simulink model "Nanosatellite"  (Simulink 10.1)
settings: Solver=FixedStepAuto  StartTime=0.0  StopTime=5  FixedStep=1e-2  RelTol=1e-3
undefined symbols (not defined in the file): a1, a2, a3, K, K1, K2, u10, u20
settings Model: Creator=NAOUE  LastModifiedBy=NAOUE
settings DataIOCC: SaveFormat=Dataset  ReturnWorkspaceOutputs=on
settings OptimizationCC: LifeSpan=auto
settings DebuggingCC: UnderspecifiedInitializationDetection=Simplified  MergeDetectMultiDrivingBlocksExec=error  SFUnexpectedBacktrackingDiag=error  SFNoUnconditionalDefaultTransitionDiag=error  SFExecutionAtInitializationDiag=warning  ArithmeticOperatorsInVariantConditions=error
settings HardwareCC: ProdBitPerPointer=64  ProdBitPerSizeT=64  ProdBitPerPtrDiffT=64  ProdLargestAtomicFloat=Float  ProdIntDivRoundTo=Zero  ProdEndianess=LittleEndian  ProdWordSize=64  ProdHWDeviceType=Intel->x86-64 (Windows64)
settings ModelReferenceCC: PropagateSignalLabelsOutOfModel=on
settings SFSimCC: SimUseLocalCustomCode=on  CustomCodeUndefinedFunction=FilterOut
settings RTWCC: RTWUseLocalCustomCode=on
settings CodeAppCC: StateflowObjectComments=off
settings GRTTargetCC: TargetLangStandard=C99 (ISO)  CombineOutputUpdateFcns=on  GRTInterface=off
settings ConfigComp: CovMetricSettings=dwe  CovHtmlReporting=off  CovSaveCumulativeToWorkspaceVar=off  CovSaveSingleToWorkspaceVar=off  CovExternalEMLEnable=on

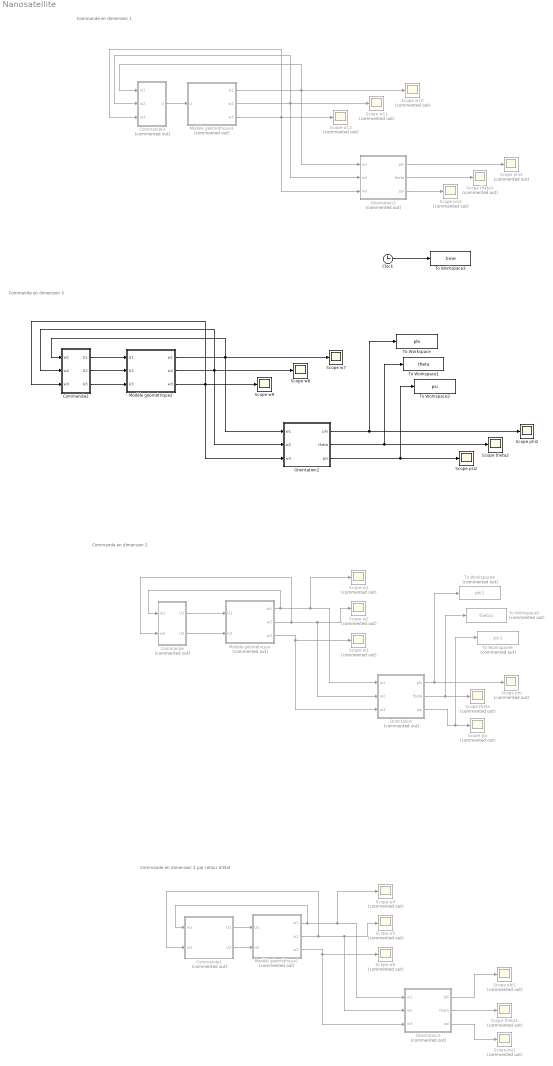
== system Nanosatellite ==
  note: Commande en dimension 2 par retour d'état
  note: Commande en dimension 2
  note: Commande en dimension 1
  note: Commande en dimension 3
  Clock : Clock
  Commande : Subsystem  Commented=on
  Commande1 : Subsystem  Commented=on
  Commande2 : Subsystem
  Commande3 : Subsystem  Commented=on
  Modèle géométrique : Subsystem  Commented=on
  Modèle géométrique1 : Subsystem  Commented=on
  Modèle géométrique2 : Subsystem
  Modèle géométrique3 : Subsystem  Commented=on
  Orientation : Subsystem  Commented=on
  Orientation1 : Subsystem  Commented=on
  Orientation2 : Subsystem
  Orientation3 : Subsystem  Commented=on
  Scope phi : Scope  Commented=on
  Scope phi1 : Scope  Commented=on
  Scope phi2 : Scope
  Scope phi3 : Scope  Commented=on
  Scope psi : Scope  Commented=on
  Scope psi1 : Scope  Commented=on
  Scope psi2 : Scope
  Scope psi3 : Scope  Commented=on
  Scope theta : Scope  Commented=on
  Scope theta1 : Scope  Commented=on
  Scope theta2 : Scope
  Scope theta3 : Scope  Commented=on
  Scope w{1..6,10..12} (9 alike) : Scope  Commented=on
  Scope w7 : Scope
  Scope w8 : Scope
  Scope w9 : Scope
  To Workspace : ToWorkspace  VariableName=phi  SampleTime=-1
  To Workspace1 : ToWorkspace  VariableName=theta  SampleTime=-1
  To Workspace2 : ToWorkspace  VariableName=psi  SampleTime=-1
  To Workspace3 : ToWorkspace  VariableName=time  SampleTime=-1
  To Workspace4 : ToWorkspace  Commented=on  VariableName=phi1  SampleTime=-1
  To Workspace5 : ToWorkspace  Commented=on  VariableName=theta1  SampleTime=-1
  To Workspace6 : ToWorkspace  Commented=on  VariableName=psi1  SampleTime=-1
  wires:
  Modèle géométrique/3(w3) -> Orientation/3(w3), Scope w3/1
  Commande/1(U1) -> Modèle géométrique/1(U1)
  Commande/2(U2) -> Modèle géométrique/2(U2)
  Modèle géométrique/1(w1) -> Commande/1(w1), Orientation/1(w1), Scope w1/1
  Modèle géométrique/2(w2) -> Commande/2(w2), Orientation/2(w2), Scope w2/1
  Modèle géométrique1/2(w2) -> Commande1/2(w2), Scope w5/1, Orientation1/2(w2)
  Modèle géométrique1/1(w1) -> Commande1/1(w1), Scope w4/1, Orientation1/1(w1)
  Commande1/2(U2) -> Modèle géométrique1/2(U2)
  Commande1/1(U1) -> Modèle géométrique1/1(U1)
  Orientation1/3(psi) -> Scope psi1/1
  Orientation1/2(theta) -> Scope theta1/1
  Orientation1/1(phi) -> Scope phi1/1
  Modèle géométrique1/3(w3) -> Scope w6/1, Orientation1/3(w3)
  Modèle géométrique2/2(w2) -> Commande2/2(w2), Scope w8/1, Orientation2/2(w2)
  Modèle géométrique2/1(w1) -> Commande2/1(w1), Scope w7/1, Orientation2/1(w1)
  Commande2/2(U2) -> Modèle géométrique2/2(U2)
  Commande2/1(U1) -> Modèle géométrique2/1(U1)
  Orientation2/3(psi) -> To Workspace2/1, Scope psi2/1
  Orientation2/2(theta) -> Scope theta2/1, To Workspace1/1
  Orientation2/1(phi) -> To Workspace/1, Scope phi2/1
  Modèle géométrique2/3(w3) -> Commande2/3(w3), Scope w9/1, Orientation2/3(w3)
  Commande2/3(U3) -> Modèle géométrique2/3(U3)
  Modèle géométrique3/3(w3) -> Orientation3/3(w3), Commande3/3(w3), Scope w12/1
  Orientation3/1(phi) -> Scope phi3/1
  Orientation3/2(theta) -> Scope theta3/1
  Orientation3/3(psi) -> Scope psi3/1
  Commande3/1(U) -> Modèle géométrique3/1(U)
  Modèle géométrique3/1(w1) -> Orientation3/1(w1), Scope w10/1, Commande3/1(w1)
  Modèle géométrique3/2(w2) -> Orientation3/2(w2), Scope w11/1, Commande3/2(w2)
  Clock/1 -> To Workspace3/1
  Orientation/1(phi) -> To Workspace4/1, Scope phi/1
  Orientation/2(theta) -> To Workspace5/1, Scope theta/1
  Orientation/3(psi) -> To Workspace6/1, Scope psi/1

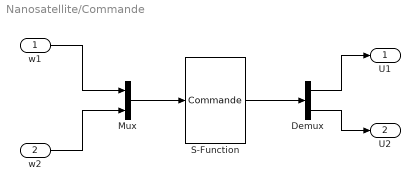
== system Nanosatellite/Commande ==
  w1 : Inport
  w2 : Inport  Port=2
  Demux : Demux  Outputs=2
  Mux : Mux  Inputs=2
  S-Function : S-Function  FunctionName=Commande  Parameters=Parametres  SFunctionDeploymentMode=off  EnableBusSupport=off
  U1 : Outport
  U2 : Outport  Port=2
  wires:
  S-Function/1 -> Demux/1
  w1/1 -> Mux/1
  Demux/1 -> U1/1
  w2/1 -> Mux/2
  Demux/2 -> U2/1
  Mux/1 -> S-Function/1

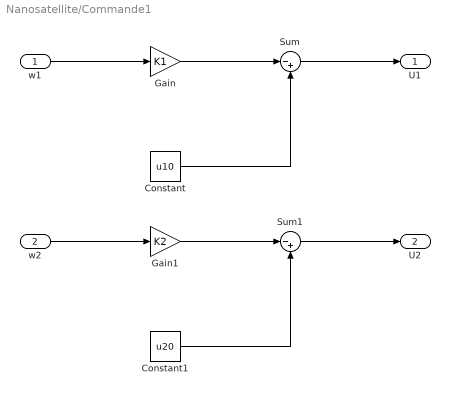
== system Nanosatellite/Commande1 ==
  w1 : Inport
  w2 : Inport  Port=2
  Constant : Constant  Value=u10
  Constant1 : Constant  Value=u20
  Gain : Gain  Gain=K1
  Gain1 : Gain  Gain=K2
  Sum : Sum  Inputs=|-+
  Sum1 : Sum  Inputs=|-+
  U1 : Outport
  U2 : Outport  Port=2
  wires:
  Gain/1 -> Sum/1
  w1/1 -> Gain/1
  Constant/1 -> Sum/2
  Sum/1 -> U1/1
  Sum1/1 -> U2/1
  Constant1/1 -> Sum1/2
  w2/1 -> Gain1/1
  Gain1/1 -> Sum1/1

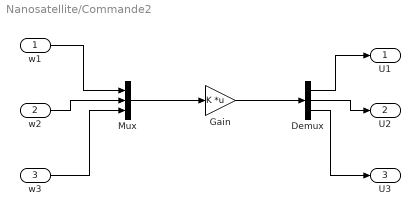
== system Nanosatellite/Commande2 ==
  w1 : Inport
  w2 : Inport  Port=2
  w3 : Inport  Port=3
  Demux : Demux  Outputs=3
  Gain : Gain  Gain=K  Multiplication=Matrix(K*u)
  Mux : Mux  Inputs=3
  U1 : Outport
  U2 : Outport  Port=2
  U3 : Outport  Port=3
  wires:
  Mux/1 -> Gain/1
  Demux/2 -> U2/1
  w2/1 -> Mux/2
  Demux/1 -> U1/1
  w1/1 -> Mux/1
  Gain/1 -> Demux/1
  w3/1 -> Mux/3
  Demux/3 -> U3/1

== system Nanosatellite/Commande3 ==
  w1 : Inport
  w2 : Inport  Port=2
  w3 : Inport  Port=3
  Mux : Mux  Inputs=3
  S-Function : S-Function  FunctionName=Commande3  SFunctionDeploymentMode=off  EnableBusSupport=off
  U : Outport
  wires:
  w3/1 -> Mux/3
  w1/1 -> Mux/1
  S-Function/1 -> U/1
  w2/1 -> Mux/2
  Mux/1 -> S-Function/1

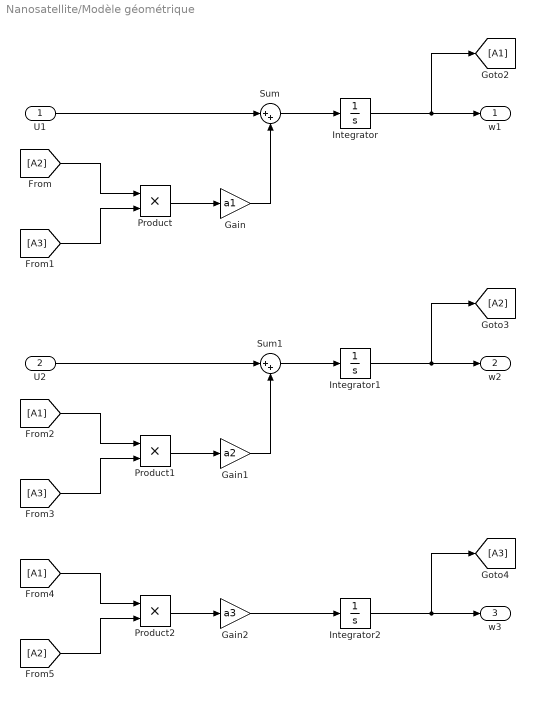
== system Nanosatellite/Modèle géométrique ==
  U1 : Inport
  U2 : Inport  Port=2
  Gain : Gain  Gain=a1
  Gain1 : Gain  Gain=a2
  Gain2 : Gain  Gain=a3
  Integrator : Integrator
  Integrator1 : Integrator
  Integrator2 : Integrator
  Product : Product
  Product1 : Product
  Product2 : Product
  Sum : Sum  Inputs=|++
  Sum1 : Sum  Inputs=|++
  w1 : Outport
  w2 : Outport  Port=2
  w3 : Outport  Port=3
  wires:
  Integrator/1 -> [A1], w1/1
  U1/1 -> Sum/1
  Sum/1 -> Integrator/1
  Gain/1 -> Sum/2
  Product/1 -> Gain/1
  [A2] -> Product/1
  [A3] -> Product/2
  [A3] -> Product1/2
  [A1] -> Product1/1
  Product1/1 -> Gain1/1
  Gain1/1 -> Sum1/2
  Sum1/1 -> Integrator1/1
  U2/1 -> Sum1/1
  Integrator1/1 -> w2/1, [A2]
  Integrator2/1 -> [A3], w3/1
  Gain2/1 -> Integrator2/1
  Product2/1 -> Gain2/1
  [A1] -> Product2/1
  [A2] -> Product2/2

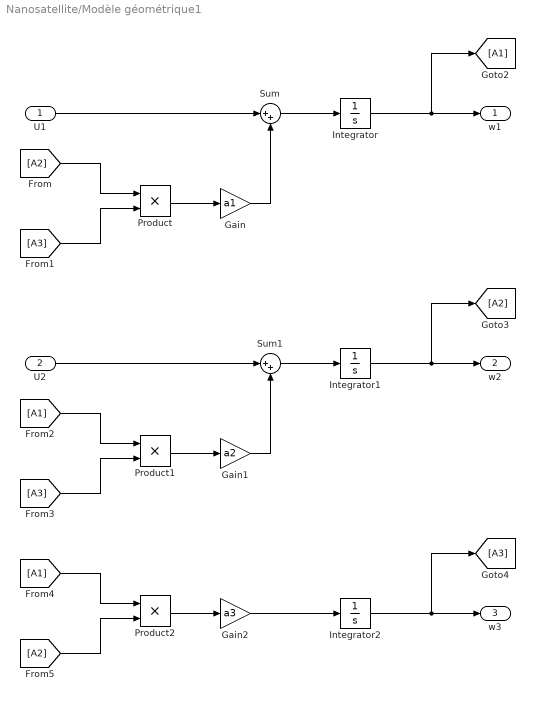
== system Nanosatellite/Modèle géométrique1 ==
  U1 : Inport
  U2 : Inport  Port=2
  Gain : Gain  Gain=a1
  Gain1 : Gain  Gain=a2
  Gain2 : Gain  Gain=a3
  Integrator : Integrator
  Integrator1 : Integrator
  Integrator2 : Integrator
  Product : Product
  Product1 : Product
  Product2 : Product
  Sum : Sum  Inputs=|++
  Sum1 : Sum  Inputs=|++
  w1 : Outport
  w2 : Outport  Port=2
  w3 : Outport  Port=3
  wires:
  [A2] -> Product2/2
  [A1] -> Product2/1
  Product2/1 -> Gain2/1
  Gain2/1 -> Integrator2/1
  Integrator2/1 -> w3/1, [A3]
  Integrator1/1 -> [A2], w2/1
  U2/1 -> Sum1/1
  Sum1/1 -> Integrator1/1
  Gain1/1 -> Sum1/2
  Product1/1 -> Gain1/1
  [A1] -> Product1/1
  [A3] -> Product1/2
  [A3] -> Product/2
  [A2] -> Product/1
  Product/1 -> Gain/1
  Gain/1 -> Sum/2
  Sum/1 -> Integrator/1
  U1/1 -> Sum/1
  Integrator/1 -> w1/1, [A1]

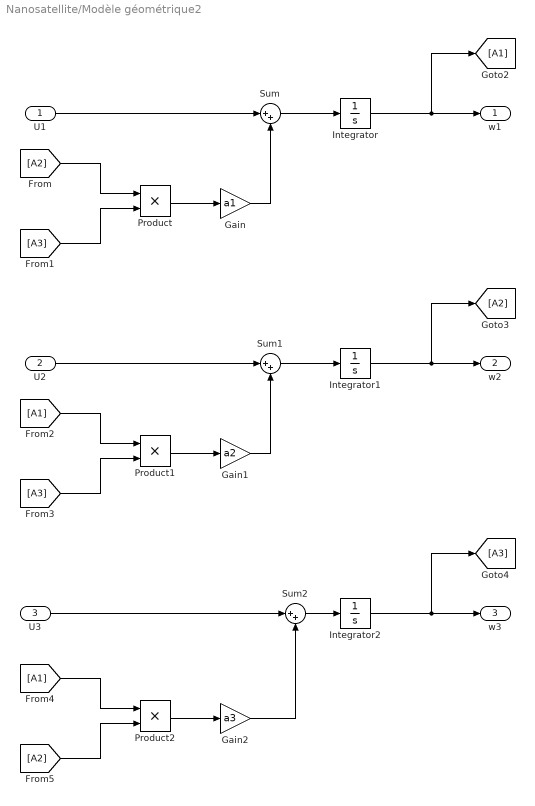
== system Nanosatellite/Modèle géométrique2 ==
  U1 : Inport
  U2 : Inport  Port=2
  U3 : Inport  Port=3
  Gain : Gain  Gain=a1
  Gain1 : Gain  Gain=a2
  Gain2 : Gain  Gain=a3
  Integrator : Integrator  InitialCondition=0.1
  Integrator1 : Integrator  InitialCondition=0.1
  Integrator2 : Integrator  InitialCondition=0.2
  Product : Product
  Product1 : Product
  Product2 : Product
  Sum : Sum  Inputs=|++
  Sum1 : Sum  Inputs=|++
  Sum2 : Sum  Inputs=|++
  w1 : Outport
  w2 : Outport  Port=2
  w3 : Outport  Port=3
  wires:
  Integrator/1 -> [A1], w1/1
  U1/1 -> Sum/1
  Sum/1 -> Integrator/1
  Gain/1 -> Sum/2
  Product/1 -> Gain/1
  [A2] -> Product/1
  [A3] -> Product/2
  [A3] -> Product1/2
  [A1] -> Product1/1
  Product1/1 -> Gain1/1
  Gain1/1 -> Sum1/2
  Sum1/1 -> Integrator1/1
  U2/1 -> Sum1/1
  Integrator1/1 -> w2/1, [A2]
  Integrator2/1 -> [A3], w3/1
  Product2/1 -> Gain2/1
  [A1] -> Product2/1
  [A2] -> Product2/2
  U3/1 -> Sum2/1
  Gain2/1 -> Sum2/2
  Sum2/1 -> Integrator2/1

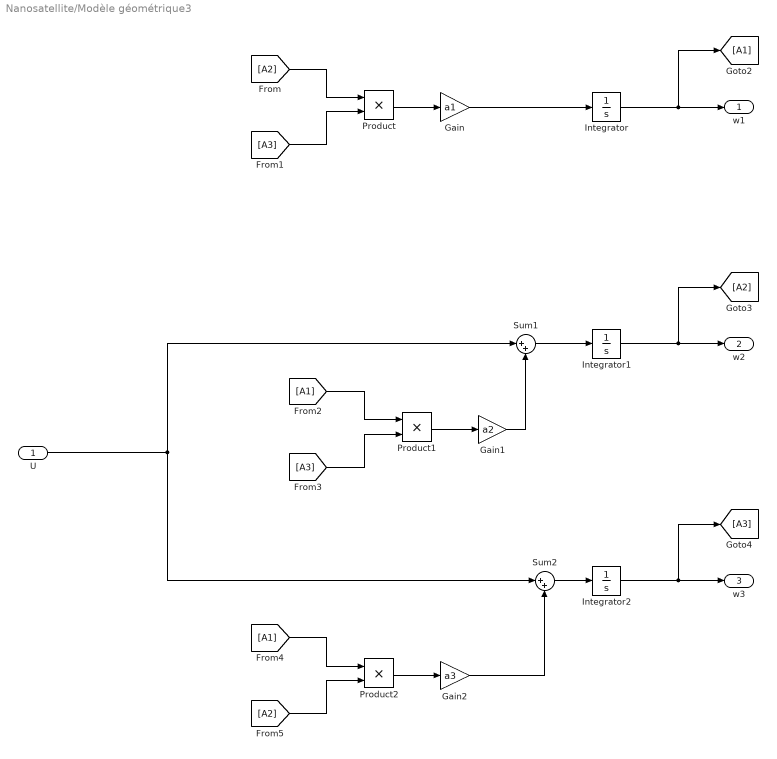
== system Nanosatellite/Modèle géométrique3 ==
  U : Inport
  Gain : Gain  Gain=a1
  Gain1 : Gain  Gain=a2
  Gain2 : Gain  Gain=a3
  Integrator : Integrator  InitialCondition=0.001
  Integrator1 : Integrator
  Integrator2 : Integrator
  Product : Product
  Product1 : Product
  Product2 : Product
  Sum1 : Sum  Inputs=|++
  Sum2 : Sum  Inputs=|++
  w1 : Outport
  w2 : Outport  Port=2
  w3 : Outport  Port=3
  wires:
  Sum2/1 -> Integrator2/1
  Gain2/1 -> Sum2/2
  [A2] -> Product2/2
  [A1] -> Product2/1
  Product2/1 -> Gain2/1
  Integrator2/1 -> w3/1, [A3]
  Integrator1/1 -> [A2], w2/1
  Sum1/1 -> Integrator1/1
  Gain1/1 -> Sum1/2
  Product1/1 -> Gain1/1
  [A1] -> Product1/1
  [A3] -> Product1/2
  [A3] -> Product/2
  [A2] -> Product/1
  Product/1 -> Gain/1
  Gain/1 -> Integrator/1
  Integrator/1 -> w1/1, [A1]
  U/1 -> Sum1/1, Sum2/1

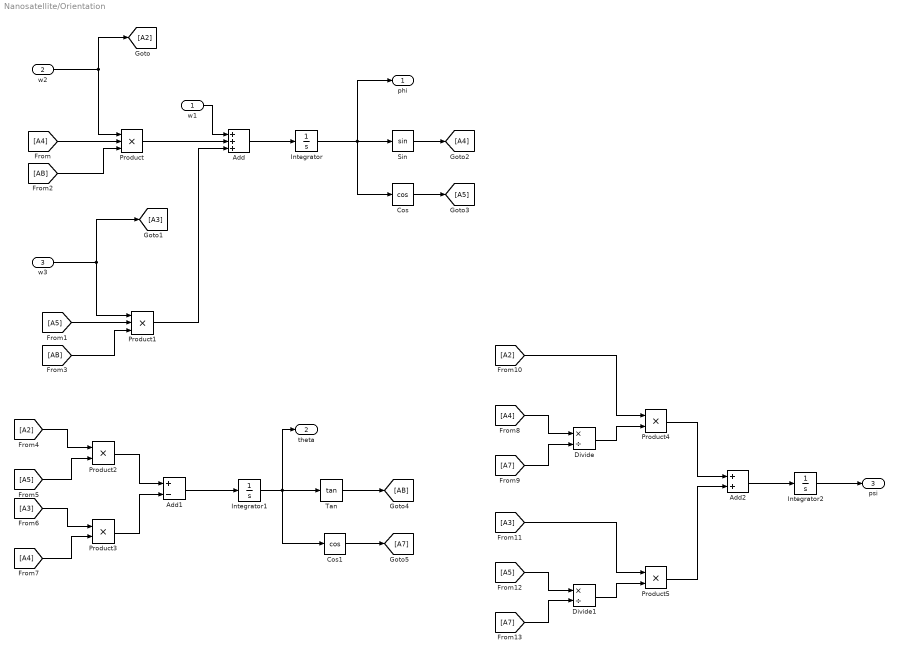
== system Nanosatellite/Orientation ==
  w1 : Inport
  w2 : Inport  Port=2
  w3 : Inport  Port=3
  Add : Sum  Inputs=+++
  Add1 : Sum  Inputs=+-
  Add2 : Sum
  Cos : Trigonometry  Operator=cos
  Cos1 : Trigonometry  Operator=cos
  Divide : Product  Inputs=*/
  Divide1 : Product  Inputs=*/
  Integrator : Integrator
  Integrator1 : Integrator
  Integrator2 : Integrator
  Product : Product  Inputs=3
  Product1 : Product  Inputs=3
  Product{2..5} (4 alike) : Product
  Sin : Trigonometry
  Tan : Trigonometry  Operator=tan
  phi : Outport
  theta : Outport  Port=2
  psi : Outport  Port=3
  wires:
  [A4] -> Product/2
  [AB] -> Product/3
  w2/1 -> [A2], Product/1
  Product/1 -> Add/2
  w1/1 -> Add/1
  Add/1 -> Integrator/1
  w3/1 -> Product1/1, [A3]
  [AB] -> Product1/3
  [A5] -> Product1/2
  Product1/1 -> Add/3
  Integrator/1 -> phi/1, Cos/1, Sin/1
  Sin/1 -> [A4]
  Cos/1 -> [A5]
  [A2] -> Product2/1
  [A5] -> Product2/2
  [A4] -> Product3/2
  [A3] -> Product3/1
  Product2/1 -> Add1/1
  Product3/1 -> Add1/2
  Add1/1 -> Integrator1/1
  Integrator1/1 -> theta/1, Cos1/1, Tan/1
  Tan/1 -> [AB]
  Cos1/1 -> [A7]
  [A7] -> Divide/2
  [A4] -> Divide/1
  [A2] -> Product4/1
  Divide/1 -> Product4/2
  Divide1/1 -> Product5/2
  [A3] -> Product5/1
  [A5] -> Divide1/1
  [A7] -> Divide1/2
  Product4/1 -> Add2/1
  Product5/1 -> Add2/2
  Add2/1 -> Integrator2/1
  Integrator2/1 -> psi/1

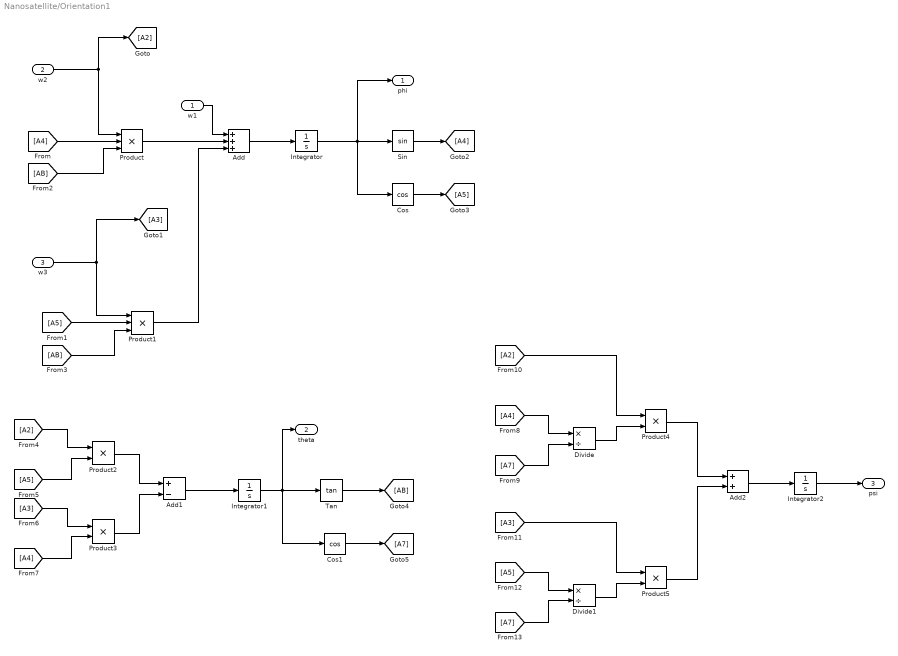
== system Nanosatellite/Orientation1 ==
  w1 : Inport
  w2 : Inport  Port=2
  w3 : Inport  Port=3
  Add : Sum  Inputs=+++
  Add1 : Sum  Inputs=+-
  Add2 : Sum
  Cos : Trigonometry  Operator=cos
  Cos1 : Trigonometry  Operator=cos
  Divide : Product  Inputs=*/
  Divide1 : Product  Inputs=*/
  Integrator : Integrator
  Integrator1 : Integrator
  Integrator2 : Integrator
  Product : Product  Inputs=3
  Product1 : Product  Inputs=3
  Product{2..5} (4 alike) : Product
  Sin : Trigonometry
  Tan : Trigonometry  Operator=tan
  phi : Outport
  theta : Outport  Port=2
  psi : Outport  Port=3
  wires:
  Integrator2/1 -> psi/1
  Add2/1 -> Integrator2/1
  Product5/1 -> Add2/2
  Product4/1 -> Add2/1
  [A7] -> Divide1/2
  [A5] -> Divide1/1
  [A3] -> Product5/1
  Divide1/1 -> Product5/2
  Divide/1 -> Product4/2
  [A2] -> Product4/1
  [A4] -> Divide/1
  [A7] -> Divide/2
  Cos1/1 -> [A7]
  Tan/1 -> [AB]
  Integrator1/1 -> Tan/1, Cos1/1, theta/1
  Add1/1 -> Integrator1/1
  Product3/1 -> Add1/2
  Product2/1 -> Add1/1
  [A3] -> Product3/1
  [A4] -> Product3/2
  [A5] -> Product2/2
  [A2] -> Product2/1
  Cos/1 -> [A5]
  Sin/1 -> [A4]
  Integrator/1 -> Sin/1, Cos/1, phi/1
  Product1/1 -> Add/3
  [A5] -> Product1/2
  [AB] -> Product1/3
  w3/1 -> [A3], Product1/1
  Add/1 -> Integrator/1
  w1/1 -> Add/1
  Product/1 -> Add/2
  w2/1 -> Product/1, [A2]
  [AB] -> Product/3
  [A4] -> Product/2

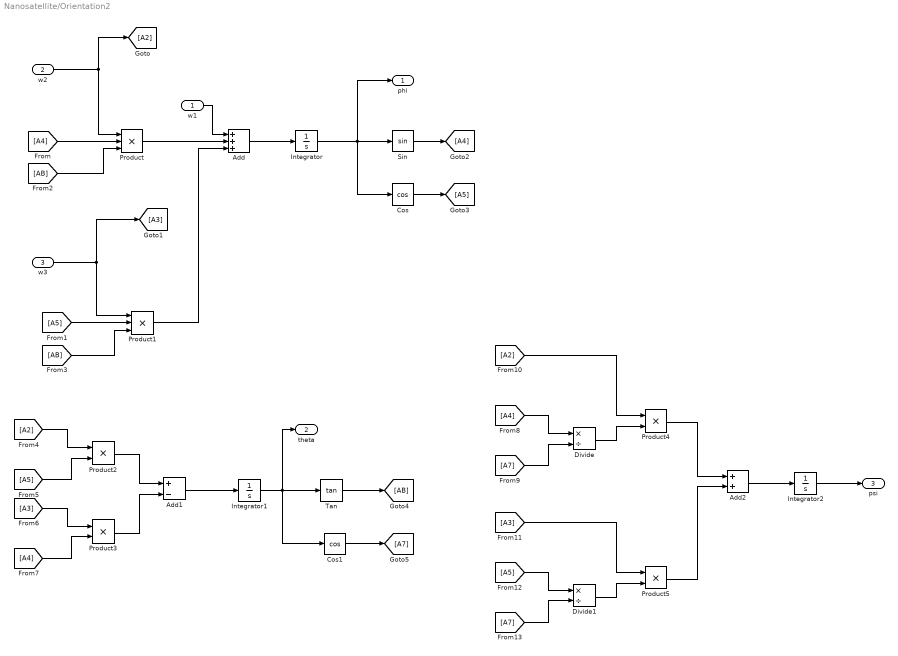
== system Nanosatellite/Orientation2 ==
  w1 : Inport
  w2 : Inport  Port=2
  w3 : Inport  Port=3
  Add : Sum  Inputs=+++
  Add1 : Sum  Inputs=+-
  Add2 : Sum
  Cos : Trigonometry  Operator=cos
  Cos1 : Trigonometry  Operator=cos
  Divide : Product  Inputs=*/
  Divide1 : Product  Inputs=*/
  Integrator : Integrator
  Integrator1 : Integrator
  Integrator2 : Integrator
  Product : Product  Inputs=3
  Product1 : Product  Inputs=3
  Product{2..5} (4 alike) : Product
  Sin : Trigonometry
  Tan : Trigonometry  Operator=tan
  phi : Outport
  theta : Outport  Port=2
  psi : Outport  Port=3
  wires:
  Integrator2/1 -> psi/1
  Add2/1 -> Integrator2/1
  Product5/1 -> Add2/2
  Product4/1 -> Add2/1
  [A7] -> Divide1/2
  [A5] -> Divide1/1
  [A3] -> Product5/1
  Divide1/1 -> Product5/2
  Divide/1 -> Product4/2
  [A2] -> Product4/1
  [A4] -> Divide/1
  [A7] -> Divide/2
  Cos1/1 -> [A7]
  Tan/1 -> [AB]
  Integrator1/1 -> Tan/1, Cos1/1, theta/1
  Add1/1 -> Integrator1/1
  Product3/1 -> Add1/2
  Product2/1 -> Add1/1
  [A3] -> Product3/1
  [A4] -> Product3/2
  [A5] -> Product2/2
  [A2] -> Product2/1
  Cos/1 -> [A5]
  Sin/1 -> [A4]
  Integrator/1 -> Sin/1, Cos/1, phi/1
  Product1/1 -> Add/3
  [A5] -> Product1/2
  [AB] -> Product1/3
  w3/1 -> [A3], Product1/1
  Add/1 -> Integrator/1
  w1/1 -> Add/1
  Product/1 -> Add/2
  w2/1 -> Product/1, [A2]
  [AB] -> Product/3
  [A4] -> Product/2

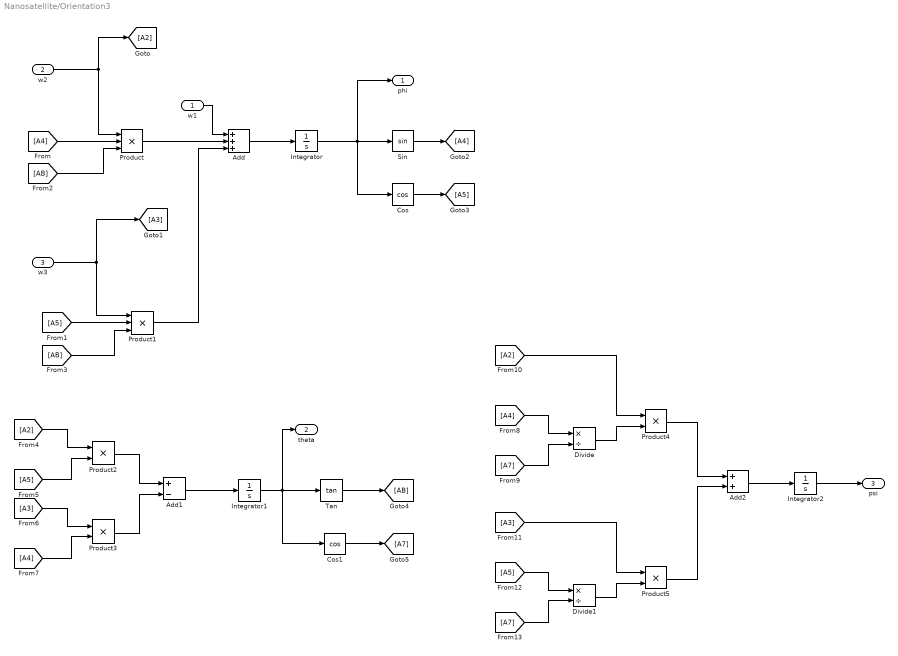
== system Nanosatellite/Orientation3 ==
  w1 : Inport
  w2 : Inport  Port=2
  w3 : Inport  Port=3
  Add : Sum  Inputs=+++
  Add1 : Sum  Inputs=+-
  Add2 : Sum
  Cos : Trigonometry  Operator=cos
  Cos1 : Trigonometry  Operator=cos
  Divide : Product  Inputs=*/
  Divide1 : Product  Inputs=*/
  Integrator : Integrator
  Integrator1 : Integrator
  Integrator2 : Integrator
  Product : Product  Inputs=3
  Product1 : Product  Inputs=3
  Product{2..5} (4 alike) : Product
  Sin : Trigonometry
  Tan : Trigonometry  Operator=tan
  phi : Outport
  theta : Outport  Port=2
  psi : Outport  Port=3
  wires:
  [A4] -> Product/2
  [AB] -> Product/3
  w2/1 -> [A2], Product/1
  Product/1 -> Add/2
  w1/1 -> Add/1
  Add/1 -> Integrator/1
  w3/1 -> Product1/1, [A3]
  [AB] -> Product1/3
  [A5] -> Product1/2
  Product1/1 -> Add/3
  Integrator/1 -> phi/1, Cos/1, Sin/1
  Sin/1 -> [A4]
  Cos/1 -> [A5]
  [A2] -> Product2/1
  [A5] -> Product2/2
  [A4] -> Product3/2
  [A3] -> Product3/1
  Product2/1 -> Add1/1
  Product3/1 -> Add1/2
  Add1/1 -> Integrator1/1
  Integrator1/1 -> theta/1, Cos1/1, Tan/1
  Tan/1 -> [AB]
  Cos1/1 -> [A7]
  [A7] -> Divide/2
  [A4] -> Divide/1
  [A2] -> Product4/1
  Divide/1 -> Product4/2
  Divide1/1 -> Product5/2
  [A3] -> Product5/1
  [A5] -> Divide1/1
  [A7] -> Divide1/2
  Product4/1 -> Add2/1
  Product5/1 -> Add2/2
  Add2/1 -> Integrator2/1
  Integrator2/1 -> psi/1
